simulink model "exp_4"  (R2013b)
settings: Solver=ode3  StartTime=0.0  StopTime=10.0  FixedStep=0.02  RelTol=1e-3
libraries: simulink x3
settings Model: Creator=lenovo  LastModifiedBy=lenovo

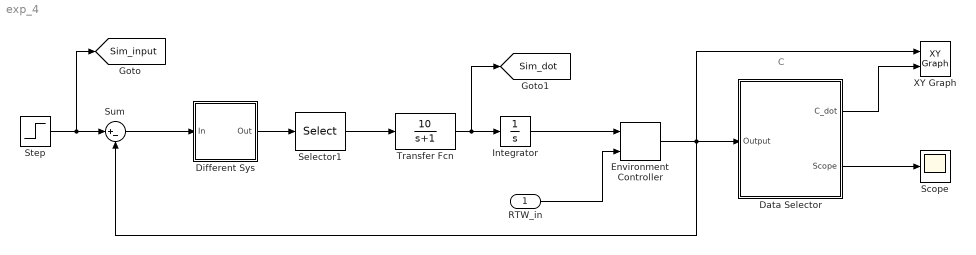
== system exp_4 ==
  note: C
  RTW_in : Inport
  "Data Selector " : Subsystem
  Different Sys : Subsystem
  Environment Controller : simulink/Signal Routing/Environment Controller
  Integrator : Integrator
  Scope : Scope
  Selector1 : Selector  InputPortWidth=4  IndexOptions=Index vector (dialog)  Indices=3  OutputSizes=1
  Step : Step  SampleTime=0
  Sum : Sum  Inputs=|+-
  Transfer Fcn : TransferFcn  Numerator=[10]  Denominator=[1 1]
  XY Graph : simulink/Sinks/XY Graph  xmin=-5  xmax=5  ymin=-5  ymax=5  st=-1
  tag scope: Sim_dot=global, Sim_input=global
  wires:
  Step/1 -> [Sim_input], Sum/1
  Sum/1 -> Different Sys/1(In)
  Different Sys/1(Out) -> Selector1/1
  Selector1/1 -> Transfer Fcn/1
  Transfer Fcn/1 -> [Sim_dot], Integrator/1
  RTW_in/1 -> Environment Controller/2
  Integrator/1 -> Environment Controller/1
  Environment Controller/1 -> Sum/2, "Data Selector "/1(Output), XY Graph/1
  "Data Selector "/1(C_dot) -> XY Graph/2
  "Data Selector "/2(Scope) -> Scope/1

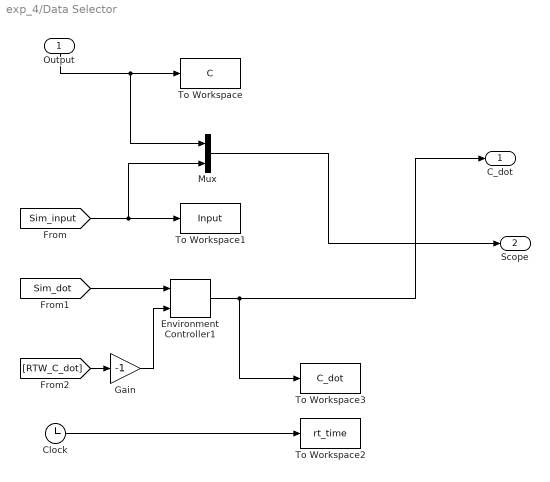
== system exp_4/Data Selector  ==
  Output : Inport
  Clock : Clock
  Environment Controller1 : simulink/Signal Routing/Environment Controller
  Gain : Gain  Gain=-1
  Mux : Mux  Inputs=2
  To Workspace : ToWorkspace  VariableName=C  SampleTime=-1  SaveFormat=Timeseries
  To Workspace1 : ToWorkspace  VariableName=Input  SampleTime=-1  SaveFormat=Timeseries
  To Workspace2 : ToWorkspace  VariableName=rt_time  SampleTime=-1  SaveFormat=Timeseries
  To Workspace3 : ToWorkspace  VariableName=C_dot  SampleTime=-1  SaveFormat=Timeseries
  C_dot : Outport
  Scope : Outport  Port=2
  wires:
  [RTW_C_dot] -> Gain/1
  [Sim_dot] -> Environment Controller1/1
  Mux/1 -> Scope/1
  Gain/1 -> Environment Controller1/2
  [Sim_input] -> Mux/2, To Workspace1/1
  Clock/1 -> To Workspace2/1
  Environment Controller1/1 -> C_dot/1, To Workspace3/1
  Output/1 -> To Workspace/1, Mux/1

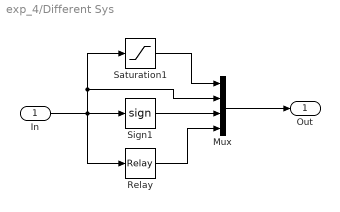
== system exp_4/Different Sys ==
  In : Inport
  Mux : Mux
  Relay : Relay
  Saturation1 : Saturate
  Sign1 : Signum
  Out : Outport
  wires:
  Saturation1/1 -> Mux/1
  Sign1/1 -> Mux/3
  Relay/1 -> Mux/4
  In/1 -> Relay/1, Sign1/1, Mux/2, Saturation1/1
  Mux/1 -> Out/1
